simulink subsystem "s_adaptive_pacing_control"  (R2024b)
settings: Solver=VariableStepAuto  StartTime=0.0  StopTime=10.0  RelTol=1e-3
undefined symbols (not defined in the file): magnitude
libraries: frdmk64flib x1
settings Model: Creator=habel  LastModifiedBy=habel

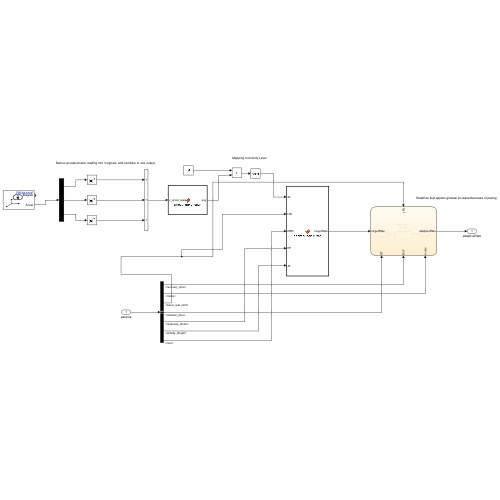
[thumbnail: Simulink's stored preview of the top-level diagram]
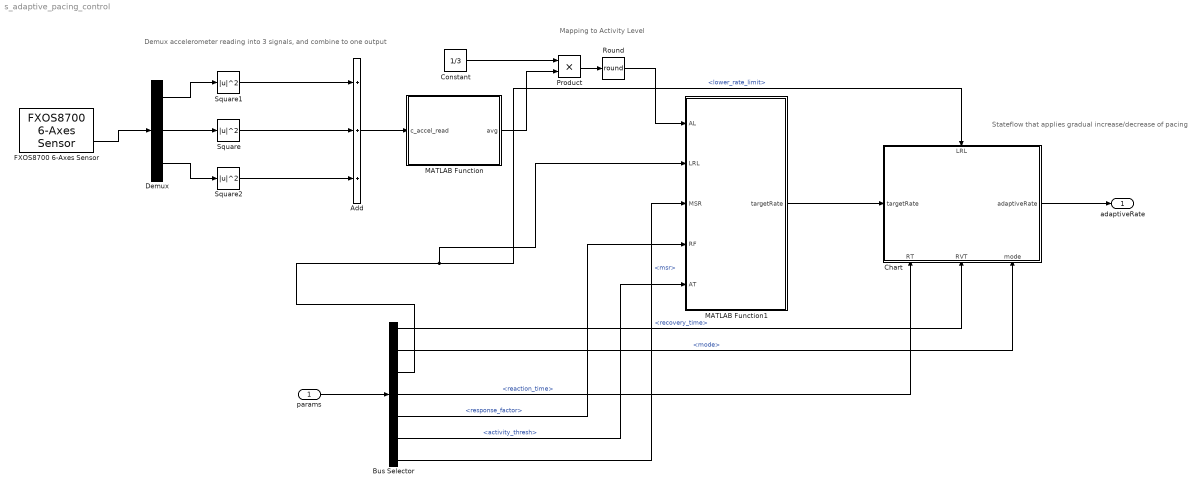
== system s_adaptive_pacing_control ==
  note: Stateflow that applies gradual increase/decrease of pacing
  note: Demux accelerometer reading into 3 signals, and combine to one output
  note: Mapping to Activity Level
  params : Inport
  Add : Sum  Inputs=+++
  Bus Selector : BusSelector  OutputSignals=recovery_time,mode,lower_rate_limit,reaction_time,response_factor,activity_thresh,msr
  Chart : Stateflow chart  TreatAsAtomicUnit=on
      settings: PortSchema="{\"entries\":[{\"content\":{\"sides\":[{\"content\":{\"connectorIds\":[\"In1\"]},\"type\":\"ConnectorPlacement.EquallySpacedRectSide\",\"uuid\":\"d0030ce2-0836-460c-8466-691187d70d9f\"},{\"content\":{\"connectorIds\":[\"Out1\"],\"side\":\"RIGHT\"},\"type\":\"ConnectorPlacement.EquallySpacedRectSide\",\"uuid\":\"9b1c10c6-cf7e-4410-bcee-8bfc88126271\"},{\"content\":{\"connectorIds\":[\"In2\"],\"side\":\"TOP\"},\"type\":\"ConnectorPlacement.EquallySpacedRectSide\",\"uuid\":\"993b59fc-6f22-431b-ad2b-b08003e60e71\"},{\"content\":{\"connectorIds\":[\"In3\",\"In4\",\"In5\"],\"side\":\"BOTTOM\"},\"type\":\"ConnectorPlacement.EquallySpacedRectSide\",\"uuid\":\"6c27a6b7-4768-4b7b-9443-aab87b8ea12c\"}]},\"type\":\"ConnectorPlacement.EquallySpacedConnector\",\"uuid\":\"fb8bcacf-49be-4bda-8c45-19ae06fb484b\"}],\"packageUris\":[\"http://schema.mathworks.com/mf0/Connector/R2020b\"],\"version\":\"1.0\"}"
  Constant : Constant  Value=1/3
  Demux : Demux  Outputs=3
  FXOS8700 6-Axes Sensor : frdmk64flib/FXOS8700 6-Axes Sensor  Activesensor=Accelerometer and Magnetometer  ODR=800Hz  HybridODR=400Hz  Accelfullrange=-4g to +4g  SampleTime=-1
  MATLAB Function : MATLAB Function  TreatAsAtomicUnit=on
  MATLAB Function1 : MATLAB Function  TreatAsAtomicUnit=on
  Product : Product
  Round : Rounding  Operator=round
  Square : Math  Operator=magnitude^2
  Square1 : Math  Operator=magnitude^2
  Square2 : Math  Operator=magnitude^2
  adaptiveRate : Outport
  wires:
  MATLAB Function1/1(targetRate) -> Chart/1(targetRate)
  Square/1 -> Add/2
  Square1/1 -> Add/1
  Constant/1 -> Product/1
  Add/1 -> MATLAB Function/1(c_accel_read)
  MATLAB Function/1(avg) -> Product/2
  Square2/1 -> Add/3
  Round/1 -> MATLAB Function1/1(AL)
  Product/1 -> Round/1
  Demux/1 -> Square1/1
  Demux/2 -> Square/1
  Demux/3 -> Square2/1
  params/1 -> Bus Selector/1
  Bus Selector/1 -> Chart/4(RVT)  "<recovery_time>"
  Bus Selector/2 -> Chart/5(mode)  "<mode>"
  Bus Selector/3 -> Chart/2(LRL), MATLAB Function1/2(LRL)  "<lower_rate_limit>"
  Bus Selector/4 -> Chart/3(RT)  "<reaction_time>"
  Bus Selector/5 -> MATLAB Function1/4(RF)  "<response_factor>"
  Bus Selector/6 -> MATLAB Function1/5(AT)  "<activity_thresh>"
  Bus Selector/7 -> MATLAB Function1/3(MSR)  "<msr>"
  Chart/1(adaptiveRate) -> adaptiveRate/1
  FXOS8700 6-Axes Sensor/2 -> Demux/1

== stateflow chart s_adaptive_pacing_control/Chart ==
  state RESET_PACE_RATE
    entry:
    adaptiveRate = double(LRL)
  state UPDATE_PACE_RATE_STEP
    entry:
    %%Compute Stepsize using Recovery Time/Reaction Time
    if adaptiveRate > targetRate
    stepSize = double(adaptiveRate - targetRate) / (double(RVT) * 60 * 1000);
    elseif adaptiveRate < targetRate
    stepSize = double((targetRate - adaptiveRate) / (double(RT) * 1000));
    else
    adaptiveRate = adaptiveRate;
    stepSize = 0.0;
    end
  state DECREASE_PACE_RATE
    entry:
    if adaptiveRate > targetRate
    adaptiveRate = adaptiveRate - stepSize;
    end
  state INCREASE_PACE_RATE
    entry:
    if adaptiveRate < targetRate
    adaptiveRate = adaptiveRate + stepSize;
    end
  (default) -> RESET_PACE_RATE
  RESET_PACE_RATE -> UPDATE_PACE_RATE_STEP : %% Adapt current rate for R modes
      | [mode > 4]
  UPDATE_PACE_RATE_STEP -> RESET_PACE_RATE [order 1] : %% Reset back to LRL for non - R modes
      | [mode < 5]
  UPDATE_PACE_RATE_STEP -> DECREASE_PACE_RATE [order 2] : %%Decrease to target
      | [adaptiveRate > targetRate]
  UPDATE_PACE_RATE_STEP -> INCREASE_PACE_RATE [order 3] : %% Increase to target
      | [adaptiveRate < targetRate]
  DECREASE_PACE_RATE -> UPDATE_PACE_RATE_STEP [order 1] : [adaptiveRate <= targetRate]
  INCREASE_PACE_RATE -> UPDATE_PACE_RATE_STEP [order 2] : %%Determine new stepsize
      | [adaptiveRate >= targetRate]
  DECREASE_PACE_RATE -> DECREASE_PACE_RATE [order 2] : after(1,msec)
  INCREASE_PACE_RATE -> INCREASE_PACE_RATE [order 1] : after(1,msec)
  data: targetRate input; LRL input; RT input; RVT input; mode input; adaptiveRate output; stepSize local

== matlab function s_adaptive_pacing_control/MATLAB Function ==
  data: c_accel_read input; avg output
%Applies a Moving Average Filter (FIR low-pass)

function avg = smoothingFunction(c_accel_read)
    %initialize storage for past samples
    persistent buffer index count; 

    N = 20; %window size of 20 samples

    %on startup, fill the buffer and initialize iterator
    if isempty(buffer) 
        buffer = zeros(1, N)
        index = 1;
        count = 0;
    end

    buffer(index) = c_accel_read; %add the recent sample to the window
    %update index circularly (shift window rightwards)
    index = mod(index, N) + 1; 

    count = min(count + 1, N); %coefficient are adjusted dynamically

    avg = sum(buffer) / count; %returns the average (smoothed output)

end

== matlab function s_adaptive_pacing_control/MATLAB Function1 ==
  data: AL input; LRL input; MSR input; targetRate output; RF input; AT input
%Maps desired pacing rate between LRL and MSR

function targetRate = desiredPacingRate(AL, LRL, MSR, RF, AT)
    % no signficant change in activity level, clamp to LRL
    if AL < AT  
        targetRate = LRL;
    else
        % apply a linear rate-transformation curve (Tutorial-4)
        targetRate = min(LRL + (AL - AT) * RF, MSR); 
    end
end
